simulink model "simulazione_non_lineare"  (R2022b)
settings: Solver=VariableStepAuto  StartTime=0.0  StopTime=100  RelTol=1e-3
settings Model: Creator=eleon  LastModifiedBy=tomma

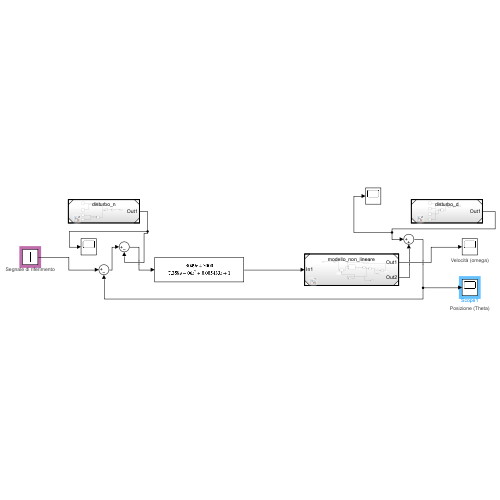
[thumbnail: Simulink's stored preview of the top-level diagram]
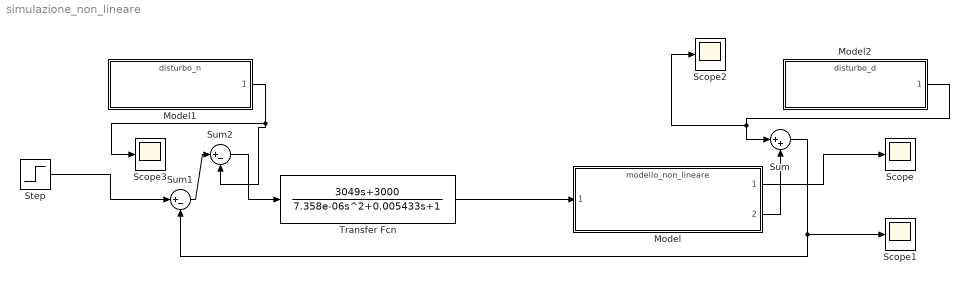
== system simulazione_non_lineare ==
  Model : ModelReference  ModelNameDialog=modello_non_lineare  UsingDefaultArgumentValue=0,0  SimulationMode=Normal  ModelReferenceVersion=1.7
  Model1 : ModelReference  ModelNameDialog=disturbo_n.slx  UsingDefaultArgumentValue=0  SimulationMode=Normal  ModelReferenceVersion=1.1
  Model2 : ModelReference  ModelNameDialog=disturbo_d  UsingDefaultArgumentValue=0  SimulationMode=Normal  ModelReferenceVersion=1.1
  Scope{,1..3} (4 alike) : Scope
      Scope settings: AttributesFormatString=Velocità (omega)
      Scope1 settings: Tag=Posizione (theta)  AttributesFormatString=Posizione (Theta)
  Step : Step  Time=0  After=10  SampleTime=0
      settings: AttributesFormatString=Segnale di riferimento
  Sum : Sum  Inputs=|++
  Sum1 : Sum  Inputs=|+-
  Sum2 : Sum  Inputs=|+-
  Transfer Fcn : TransferFcn  Numerator=[3049 3000]  Denominator=[7.358e-06 0.005433 1]
  wires:
  Model/1 -> Scope/1
  Model/2 -> Sum/2
  Transfer Fcn/1 -> Model/1
  Sum1/1 -> Sum2/1
  Model1/1 -> Scope3/1, Sum2/2
  Sum2/1 -> Transfer Fcn/1
  Model2/1 -> Scope2/1, Sum/1
  Step/1 -> Sum1/1
  Sum/1 -> Sum1/2, Scope1/1
